simulink model "uwb_hw_cosim_kintex"  (Simulink 8.0)
settings: Solver=ode45  StartTime=0.0  StopTime=33  RelTol=1e-3
InitFcn:
  | clear
  | %set_channel;
  | load channel;
  | Int_Data_input;
StopFcn:
  | bit_to_dec_excel;
  | abc=1;
values from neighbouring files (symbols this model uses):
  bit_rate = 9.7656e5    (= 976560)    [Int_Data_input.m]
undefined symbols (not defined in the file or in its folder): rsgenpoly
libraries: commutil2 x88, simulink x53, dspmtrx3 x32, dspindex x16, commcnvcod2 x8, commblkcod2 x8, dspsigops x3, commsink2 x2, xbsIndex_r4 x1, commchan3 x1, JTAGRuntimeCosim_r4 x1
(part 1 of 5)
settings Model: Creator=minhtu  LastModifiedBy=Administrator
settings DataIOCC: SignalLoggingSaveFormat=ModelDataLogs
settings DebuggingCC: FcnCallInpInsideContextMsg=UseLocalSettings
settings CodeAppCC: CustomSymbolStrType=$N$R$M_T  InternalIdentifier=Shortened
settings GRTTargetCC: CombineOutputUpdateFcns=off  GRTInterface=on

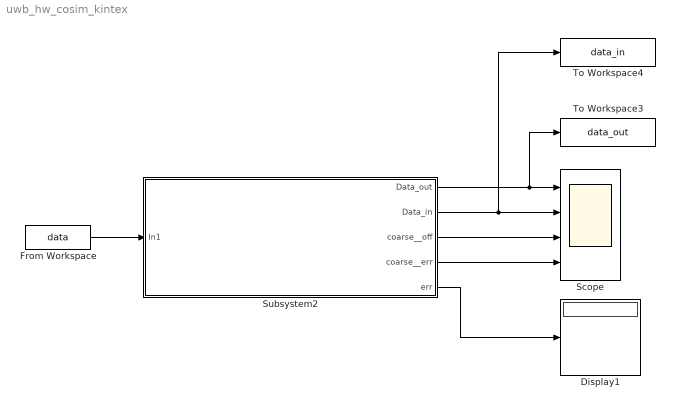
== system uwb_hw_cosim_kintex ==
  Display1 : Display
  From Workspace : FromWorkspace  VariableName=data  SampleTime=1/100
  Scope : Scope  NumInputPorts=4
      settings: YMin=0~0~1~-5  YMax=1~1~1~5  MaxDataPoints=50000000
  Subsystem2 : Subsystem
      mask Display:
      | disp('UWB_SYSTEM')
      | port_label('input',1,'data_in');
      | port_label('output',1,'data_out');
      | port_label('output',2,'data_in_delay');
      | port_label('output',3,'coarse_off');
      | port_label('output',4,'coarse_err');
      | port_label('output',5,'err');
  To Workspace3 : ToWorkspace  VariableName=data_out  SampleTime=1/100  SaveFormat=Structure
  To Workspace4 : ToWorkspace  VariableName=data_in  SampleTime=1/100  SaveFormat=Structure
  wires:
  From Workspace/1 -> Subsystem2/1(In1)
  Subsystem2/1(Data_out) -> To Workspace3/1, Scope/1
  Subsystem2/2(Data_in) -> To Workspace4/1, Scope/2
  Subsystem2/5(err) -> Display1/1
  Subsystem2/3(coarse__off) -> Scope/3
  Subsystem2/4(coarse__err) -> Scope/4

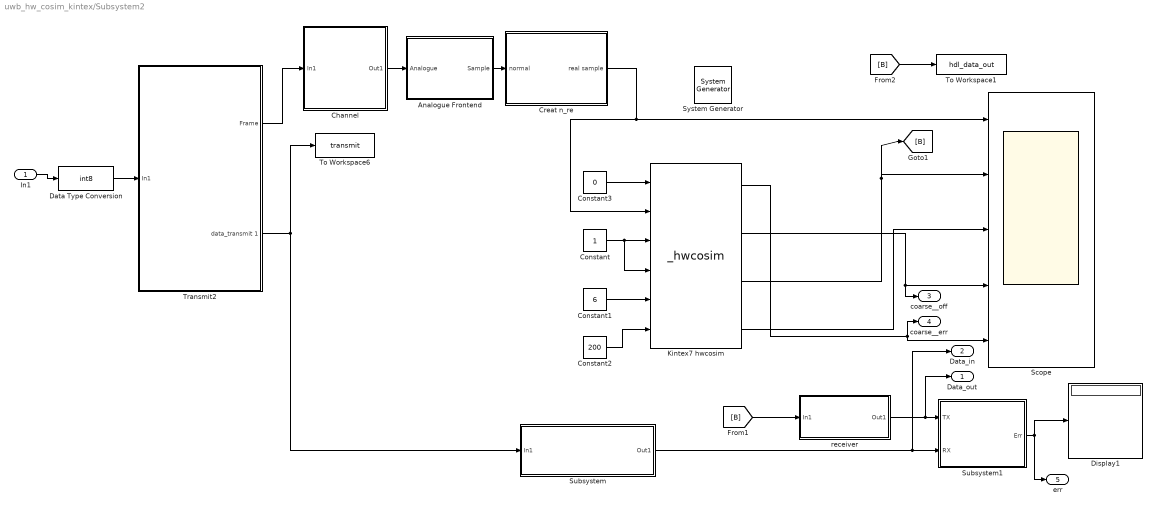
== system uwb_hw_cosim_kintex/Subsystem2 ==
  In1 : Inport
  " System Generator" : xbsIndex_r4/ System Generator  Tag=genX  xilinxfamily=kintex7  part=xc7k325t  speed=-2  package=ffg900  synthesis_tool=XST  clock_wrapper=Clock Enables  directory=./netlist  proj_type=Project Navigator  Synth_file=XST Defaults  Impl_file=ISE Defaults  testbench=off  simulink_period=3.3/31488  sysclk_period=20  dcm_input_clock_period=10  incr_netlist=off  trim_vbits=Everywhere in SubSystem  dbl_ovrd=According to Block Masks  core_generation=According to Block Masks  run_coregen=off  deprecated_control=off  eval_field=0  block_type=sysgen
  Analogue Frontend : Subsystem
  Channel : Subsystem
      mask Display: disp('CHANNEL')
  Constant : Constant
  Constant1 : Constant  Value=6
  Constant2 : Constant  Value=200
  Constant3 : Constant  Value=0
  Creat n_re : Subsystem
  Data Type Conversion : DataTypeConversion  OutDataTypeStr=int8  SampleTime=1/100
  Display1 : Display
  Kintex7 hwcosim : JTAGRuntimeCosim_r4/_hwcosim  clkSrc=Single Stepped  hasCombinationalPath=on  bitfileName=D:/z_WORKSPACE/UWB/uwb_implementation_final_kintex_final/netlist/subsystem2_cw.bit  skipConfig=off  cable=Xilinx Platform USB  speed=12 MHz  cablePort=USB21  cableParameters=xilinx_platformusb port=USB21 frequency=12000000  cableLocation=Local  shareCable=off  enable_codebug=on  savedCableParameters=xilinx_platformusb port=USB21 frequency=12000000  design_xtable=|  engineDll=JTAGCosimEngine.dll  cableWaitTime=10  bscanPos=-1  IRLengths=[]  useWaitBox=1  hasBufgmux=on  Scheme=Cosim  useCmdProc=1  hasProc=0  useImpact=0  printLogFile=0  block_type=jtagcosim
      | {
      |   'clkWrapper' => 'subsystem2_cw',
      |   'clocksGcd' => 1,
      |   'device' => 'xc7k325t-2ffg900',
      |   'ports' => {
      |     'coarse_error' => {
      |       'bd_port_index' => 0,
      |       'direction' => 'out',
      |       'icon_text' => 'coarse_error',
      |       'period' => 1,
      |       'sim_pause_trigger' => false,
      |       'type' => 'UFix_1_0',
      |       'width' => 1,
      |     },
      |     'coarse_off' => {
      |       'bd_port_index' => 1,
      |       'direction' => 'out',
      |       'icon_text' => 'coarse_off',
      |       'period' => 1,
      |       'sim_pause_trigger' => false,
      |       'type' => 'UFix_1_0',
      |       'width' => 1,
      |     },
      |     'data_out' => {
      |       'bd_port_index' => 2,
      |       'direction' => 'out',
      |       'icon_text' => 'data_out',
      |       'period' => 1,
      |       'sim_pause_trigger' => false,
      |       'type' => 'UFix_1_0',
      |       'width' => 1,
      |     },
      |     'ddph_i' => {
      |       'bd_port_index' => 0,
      |       'direction' => 'in',
      |       'icon_text' => 'ddph_i',
      |       'period' => 1,
      |       'sim_pause_trigger' => false,
      |       'type' => 'UFix_3_0',
      |       'width' => 3,
      |     },
      |     'in_data' => {
      |       'bd_port_index' => 1,
      |       'direction' => 'in',
      |       'icon_text' => 'in_data',
      |       'period' => 1,
      |       'sim_pause_trigger' => false,
      |       'type' => 'UFix_8_0',
      |       'width' => 8,
      |     },
      |     'in_rst' => {
      |       'bd_port_index' => 2,
      |       'direction' => 'in',
      |       'icon_text' => 'in_rst',
      |       'period' => 1,
      |       'sim_pause_trigger' => false,
      |       'type' => 'UFix_1_0',
      |       'width' => 1,
      |     },
      |     'in_start' => {
      |       'bd_port_index' => 3,
      |       'direction' => 'in',
      |       'icon_text' => 'in_start',
      |       'period' => 1,
      |       'sim_pause_trigger' => false,
      |       'type' => 'UFix_1_0',
      |       'width' => 1,
      |     },
      |     'psdu_en' => {
      |       'bd_port_index' => 3,
      |       'direction' => 'out',
      |       'icon_text' => 'psdu_en',
      |       'period' => 1,
      |       'sim_pause_trigger' => false,
      |       'type' => 'UFix_1_0',
      |       'width' => 1,
      |     },
      |     'sfd_threshold' => {
      |       'bd_port_index' => 4,
      |       'direction' => 'in',
      |       'icon_text' => 'sfd_threshold',
      |       'period' => 1,
      |       'sim_pause_trigger' => false,
      |       'type' => 'UFix_32_0',
      |       'width' => 32,
      |     },
      |     'sm_threshold' => {
      |       'bd_port_index' => 5,
      |       'direction' => 'in',
      |       'icon_text' => 'sm_threshold',
      |       'period' => 1,
      |       'sim_pause_trigger' => false,
      |       'type' => 'UFix_16_0',
      |       'width' => 16,
      |     },
      |   },
      |   'shared_memories' => {},
      | }
  Scope : Scope  NumInputPorts=5
      settings: TimeRange=33  YMin=0~0~0~0~0  YMax=300~1~1~1~1  MaxDataPoints=2000000
  Subsystem : Subsystem
      mask Display: disp('Delay_Data');
  Subsystem1 : Subsystem
      mask Display:
      | disp('Error Rate\n \n')
      | disp('Caculation')
      | port_label('input',1,'Rx');
      | port_label('input',2,'Tx');
      | port_label('output',1,'Err');
  To Workspace1 : ToWorkspace  VariableName=hdl_data_out  SampleTime=3.3/492  SaveFormat=Structure
  To Workspace6 : ToWorkspace  VariableName=transmit  SampleTime=3.3  SaveFormat=Structure
  Transmit2 : Subsystem
  receiver : Subsystem
      mask Display: disp('Rec_bit')
  Data_out : Outport
  Data_in : Outport  Port=2
  coarse__off : Outport  Port=3
  coarse__err : Outport  Port=4
  err : Outport  Port=5
  wires:
  Subsystem1/1(Err) -> err/1, Display1/1
  [B] -> receiver/1(In1)
  Transmit2/1(Frame) -> Channel/1(In1)
  Channel/1(Out1) -> Analogue Frontend/1(Analogue)
  Analogue Frontend/1(Sample) -> Creat n_re/1(normal)
  Kintex7 hwcosim/3 -> [B], Scope/2
  Kintex7 hwcosim/4 -> Scope/3
  Kintex7 hwcosim/2 -> coarse__off/1, Scope/4
  Kintex7 hwcosim/1 -> coarse__err/1, Scope/5
  [B] -> To Workspace1/1
  Creat n_re/1(real sample) -> Kintex7 hwcosim/2, Scope/1
  Constant3/1 -> Kintex7 hwcosim/1
  Transmit2/2(data_transmit 1) -> To Workspace6/1, Subsystem/1(In1)
  Subsystem/1(Out1) -> Data_in/1, Subsystem1/2(RX)
  Data Type Conversion/1 -> Transmit2/1(In1)
  receiver/1(Out1) -> Data_out/1, Subsystem1/1(TX)
  In1/1 -> Data Type Conversion/1
  Constant/1 -> Kintex7 hwcosim/4, Kintex7 hwcosim/3
  Constant1/1 -> Kintex7 hwcosim/5
  Constant2/1 -> Kintex7 hwcosim/6

== system uwb_hw_cosim_kintex/Subsystem2/Analogue Frontend ==
  note: Sample : 16 ns
  Analogue : Inport
  16 ns : Sum  Inputs=+  OutDataTypeStr=double
  Buffer : Buffer  N=32  TreatMby1Signals=One channel
  Product : Product  RndMeth=Zero
  Sample : Outport
  wires:
  Product/1 -> Buffer/1
  Buffer/1 -> 16 ns/1
  Analogue/1 -> Product/1, Product/2
  16 ns/1 -> Sample/1

== system uwb_hw_cosim_kintex/Subsystem2/Channel ==
  note: Channel CM1
  In1 : Inport
  AWGN Channel2 : commchan3/AWGN Channel  InputProcessing=Inherited (this choice will be removed - see release notes)  seed=0  noiseMode="Signal to noise ratio  (SNR)"  EbNodB=10  EsNodB=10  SNRdB=10  bitsPerSym=1  Ps=1  Tsym=1  variance=1
  Constant : Constant  Value=0  SampleTime=-1
  Counter Limited : simulink/Sources/Counter Limited  uplimit=10000000000000000  tsamp=3.3/1007616
  Data Type Conversion1 : DataTypeConversion  OutDataTypeStr=double
  Discrete FIR Filter : DiscreteFir  CoefSource=Input port  ProductDataTypeStr=int32  AccumDataTypeStr=int32  OutDataTypeStr=int32
  From Workspace3 : FromWorkspace  VariableName=delay  SampleTime=3.3/1007616  Interpolate=off  OutputAfterFinalValue=Cyclic repetition
  From File : FromFile  FileName=kenh.mat
  Gain1 : Gain  Gain=2^-3
  Relational Operator : RelationalOperator  Operator=<=  OutDataTypeStr=boolean
  delay_line : Subsystem
  Out1 : Outport
  wires:
  From File/1 -> Discrete FIR Filter/2
  Discrete FIR Filter/1 -> delay_line/1(data)
  Counter Limited/1 -> Relational Operator/1
  From Workspace3/1 -> Relational Operator/2
  Relational Operator/1 -> delay_line/3(sel)
  Constant/1 -> delay_line/2(loss_data)
  delay_line/1(data_out) -> AWGN Channel2/1
  In1/1 -> Gain1/1
  Data Type Conversion1/1 -> Discrete FIR Filter/1
  Gain1/1 -> Data Type Conversion1/1
  AWGN Channel2/1 -> Out1/1

== system uwb_hw_cosim_kintex/Subsystem2/Creat n_re ==
  normal : Inport
  Counter Limited2 : simulink/Sources/Counter Limited  uplimit=1000000000000  tsamp=3.3/31488
  Data Type Conversion : DataTypeConversion  OutDataTypeStr=uint8
  Delay : Constant  Value=84  OutDataTypeStr=double  SampleTime=3.3
  L_tpr4 : Constant  Value=0  VectorParams1D=off  OutDataTypeStr=double  SampleTime=-1
  Relational Operator1 : RelationalOperator  Operator=<=  OutDataTypeStr=boolean
  Remove 2 first error frames1 : Subsystem
  To Workspace : ToWorkspace  VariableName=delay  SampleTime=3.3  SaveFormat=Structure
  To Workspace3 : ToWorkspace  VariableName=Loss  SampleTime=3.3  SaveFormat=Structure
  Unbuffer : Unbuffer  SampleBasedProcessing=Same as frame based
  delay transmition : Subsystem
  n_re : Constant  Value=randi([31488,41408],1,1)  VectorParams1D=off  OutDataTypeStr=int32
  real sample : Outport
  wires:
  Relational Operator1/1 -> Remove 2 first error frames1/3(sel)
  n_re/1 -> Relational Operator1/1, To Workspace3/1
  L_tpr4/1 -> Remove 2 first error frames1/1(Zeros)
  Unbuffer/1 -> Remove 2 first error frames1/2(Sample)
  Counter Limited2/1 -> Relational Operator1/2
  Remove 2 first error frames1/1(data_out) -> delay transmition/1(data)
  normal/1 -> Unbuffer/1
  delay transmition/1(data_out) -> Data Type Conversion/1
  Delay/1 -> delay transmition/2(delay), To Workspace/1
  Data Type Conversion/1 -> real sample/1

== system uwb_hw_cosim_kintex/Subsystem2/Subsystem ==
  In1 : Inport
  Data Type Conversion2 : DataTypeConversion  OutDataTypeStr=double  SampleTime=1/100
  Delay : dspsigops/Delay  dly_unit=Samples  delay=495*2+2  ic_detail=off  dif_ic_for_ch=off  dif_ic_for_dly=off  ic=0  reset_popup=None
  Out1 : Outport
  wires:
  In1/1 -> Data Type Conversion2/1
  Data Type Conversion2/1 -> Delay/1
  Delay/1 -> Out1/1

== system uwb_hw_cosim_kintex/Subsystem2/Subsystem1 ==
  TX : Inport
  RX : Inport  Port=2
  Compare To Zero : simulink/Logic and Bit Operations/Compare To Zero  relop=>  OutDataTypeStr=uint8  ZeroCross=off
  Constant : Constant  Value=bit_rate
  Delay : dspsigops/Delay  dly_unit=Samples  delay=1  ic_detail=off  dif_ic_for_ch=off  dif_ic_for_dly=off  ic=0  reset_popup=None
  Delay1 : dspsigops/Delay  dly_unit=Samples  delay=992  ic_detail=off  dif_ic_for_ch=off  dif_ic_for_dly=off  ic=0  reset_popup=None
  Enabled Subsystem : Subsystem  TreatAsAtomicUnit=on
  Enabled Subsystem1 : Subsystem  TreatAsAtomicUnit=on
  Error Rate Calculation : commsink2/Error Rate Calculation  N=0  st_delay=992  cp_mode=Entire frame  subframe=[]  PMode=Port  WsName=ErrorVec  RsMode2=off  stop=off  numErr=100  maxBits=1e6
  Error Rate Calculation1 : commsink2/Error Rate Calculation  N=0  st_delay=992  cp_mode=Entire frame  subframe=[]  PMode=Port  WsName=ErrorVec  RsMode2=off  stop=off  numErr=100  maxBits=1e6
  Logical Operator1 : Logic  Operator=NOT  AllPortsSameDT=off  OutDataTypeStr=boolean
  Matrix Concatenate : Concatenate  Mode=Multidimensional array
  Merge : Merge
  Relational Operator : RelationalOperator  OutDataTypeStr=boolean
  Submatrix : dspmtrx3/Submatrix  RowSpan=One row  RowStartMode=Index  RowStartIndex=2  RowEndMode=Last  RowEndIndex=1  ColSpan=One column  ColStartMode=First  ColStartIndex=1  ColEndMode=Last  ColEndIndex=1
  Submatrix2 : dspmtrx3/Submatrix  RowSpan=One row  RowStartMode=Index  RowStartIndex=2  RowEndMode=Last  RowEndIndex=1  ColSpan=One column  ColStartMode=First  ColStartIndex=1  ColEndMode=Last  ColEndIndex=1
  Err : Outport
  wires:
  Error Rate Calculation/1 -> Enabled Subsystem1/1(In1), Submatrix/1
  Delay/1 -> Error Rate Calculation1/2
  Relational Operator/1 -> Compare To Zero/1
  Compare To Zero/1 -> Logical Operator1/1, Enabled Subsystem/Enable
  Enabled Subsystem1/1(Out1) -> Merge/1
  Submatrix/1 -> Relational Operator/1
  Merge/1 -> Matrix Concatenate/1
  Submatrix2/1 -> Relational Operator/2
  Enabled Subsystem/1(Out1) -> Merge/2
  TX/1 -> Error Rate Calculation1/1, Error Rate Calculation/1
  RX/1 -> Delay/1, Error Rate Calculation/2
  Logical Operator1/1 -> Enabled Subsystem1/Enable
  Error Rate Calculation1/1 -> Enabled Subsystem/1(In1), Submatrix2/1
  Constant/1 -> Delay1/1
  Delay1/1 -> Matrix Concatenate/2
  Matrix Concatenate/1 -> Err/1

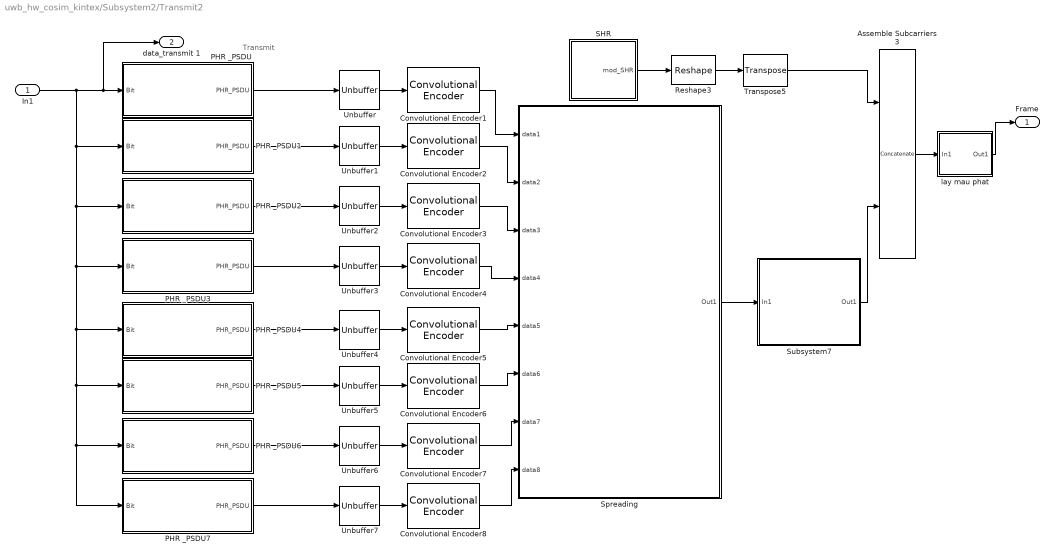
== system uwb_hw_cosim_kintex/Subsystem2/Transmit2 ==
  note: Transmit
  In1 : Inport
  Assemble Subcarriers3 : Concatenate  Mode=Multidimensional array
  Convolutional Encoder{1..8} (8 alike) : commcnvcod2/Convolutional Encoder  trellis=poly2trellis(3,[2 5])  opMode=Truncated (reset every frame)  DelayedResetAction=off  hasIniStPort=off  hasFinStPort=off  usePuncVector=off  punctureVector=[1; 1; 0; 1; 0; 1]  reset=Unused parameter value
  PHR _PSDU : Subsystem
  PHR _PSDU1 : Subsystem
  PHR _PSDU2 : Subsystem
  PHR _PSDU3 : Subsystem
  PHR _PSDU4 : Subsystem
  PHR _PSDU5 : Subsystem
  PHR _PSDU6 : Subsystem
  PHR _PSDU7 : Subsystem
  Reshape3 : Reshape  OutputDimensionality=Customize  OutputDimensions=[5,5952*32]
  SHR : Subsystem
  Spreading : Subsystem
  Subsystem7 : Subsystem
      mask Display: disp('data trc SHR');
  Transpose5 : dspmtrx3/Transpose  Hermitian=off  overflowFlag=off
  Unbuffer{,1..7} (8 alike) : Unbuffer
  lay mau phat : Subsystem
      mask Display: disp('sample')
  Frame : Outport
  data_transmit 1 : Outport  Port=2
  wires:
  Spreading/1(Out1) -> Subsystem7/1(In1)
  Convolutional Encoder4/1 -> Spreading/4(data4)
  Convolutional Encoder3/1 -> Spreading/3(data3)
  Convolutional Encoder2/1 -> Spreading/2(data2)
  Convolutional Encoder1/1 -> Spreading/1(data1)
  Unbuffer3/1 -> Convolutional Encoder4/1
  PHR _PSDU3/1(PHR_PSDU) -> Unbuffer3/1
  Unbuffer2/1 -> Convolutional Encoder3/1
  PHR _PSDU2/1(PHR_PSDU) -> Unbuffer2/1
  Unbuffer1/1 -> Convolutional Encoder2/1
  PHR _PSDU1/1(PHR_PSDU) -> Unbuffer1/1
  lay mau phat/1(Out1) -> Frame/1
  Transpose5/1 -> Assemble Subcarriers3/1
  SHR/1(mod_SHR) -> Reshape3/1
  Reshape3/1 -> Transpose5/1
  Assemble Subcarriers3/1 -> lay mau phat/1(In1)
  Subsystem7/1(Out1) -> Assemble Subcarriers3/2
  Unbuffer/1 -> Convolutional Encoder1/1
  PHR _PSDU/1(PHR_PSDU) -> Unbuffer/1
  Unbuffer7/1 -> Convolutional Encoder8/1
  PHR _PSDU7/1(PHR_PSDU) -> Unbuffer7/1
  In1/1 -> PHR _PSDU6/1(Bit), PHR _PSDU7/1(Bit), PHR _PSDU5/1(Bit), PHR _PSDU4/1(Bit), PHR _PSDU3/1(Bit), PHR _PSDU2/1(Bit), PHR _PSDU1/1(Bit), data_transmit 1/1, PHR _PSDU/1(Bit)
  Unbuffer6/1 -> Convolutional Encoder7/1
  PHR _PSDU6/1(PHR_PSDU) -> Unbuffer6/1
  Unbuffer5/1 -> Convolutional Encoder6/1
  PHR _PSDU5/1(PHR_PSDU) -> Unbuffer5/1
  Unbuffer4/1 -> Convolutional Encoder5/1
  PHR _PSDU4/1(PHR_PSDU) -> Unbuffer4/1
  Convolutional Encoder5/1 -> Spreading/5(data5)
  Convolutional Encoder6/1 -> Spreading/6(data6)
  Convolutional Encoder7/1 -> Spreading/7(data7)
  Convolutional Encoder8/1 -> Spreading/8(data8)

== system uwb_hw_cosim_kintex/Subsystem2/receiver ==
  In1 : Inport
  Buffer : Buffer  N=492  TreatMby1Signals=One channel
  Data Type Conversion2 : DataTypeConversion  OutDataTypeStr=double  SampleTime=3.3/492
  Submatrix : dspmtrx3/Submatrix  RowSpan=Range of rows  RowStartMode=Index  RowStartIndex=113  RowEndMode=Index  RowEndIndex=442  ColSpan=One column  ColStartMode=First  ColStartIndex=1  ColEndMode=Last  ColEndIndex=1
  Unbuffer : Unbuffer  SampleBasedProcessing=Same as frame based
  Out1 : Outport
  wires:
  In1/1 -> Data Type Conversion2/1
  Unbuffer/1 -> Out1/1
  Submatrix/1 -> Unbuffer/1
  Buffer/1 -> Submatrix/1
  Data Type Conversion2/1 -> Buffer/1

== system uwb_hw_cosim_kintex/Subsystem2/Channel/delay_line ==
  data : Inport
  loss_data : Inport  Port=2
  sel : Inport  Port=3
  Compare To Zero : simulink/Logic and Bit Operations/Compare To Zero  relop===  OutDataTypeStr=uint8  ZeroCross=off
  Enabled Subsystem : Subsystem  TreatAsAtomicUnit=on
  Enabled Subsystem1 : Subsystem  TreatAsAtomicUnit=on
  Logical Operator : Logic  Operator=NOT  AllPortsSameDT=off  OutDataTypeStr=boolean
  Merge : Merge
  data_out : Outport
  wires:
  loss_data/1 -> Enabled Subsystem/1(In1)
  Merge/1 -> data_out/1
  sel/1 -> Compare To Zero/1
  data/1 -> Enabled Subsystem1/1(In1)
  Compare To Zero/1 -> Logical Operator/1, Enabled Subsystem1/Enable
  Enabled Subsystem1/1(Out1) -> Merge/1
  Enabled Subsystem/1(Out1) -> Merge/2
  Logical Operator/1 -> Enabled Subsystem/Enable

== system uwb_hw_cosim_kintex/Subsystem2/Creat n_re/Remove 2 first error frames1 ==
  Zeros : Inport
  Sample : Inport  Port=2
  sel : Inport  Port=3
  Compare To Zero : simulink/Logic and Bit Operations/Compare To Zero  relop===  OutDataTypeStr=uint8  ZeroCross=off
  Enabled Subsystem : Subsystem  TreatAsAtomicUnit=on
  Enabled Subsystem1 : Subsystem  TreatAsAtomicUnit=on
  Logical Operator : Logic  Operator=NOT  AllPortsSameDT=off  OutDataTypeStr=boolean
  Merge : Merge
  data_out : Outport
  wires:
  Sample/1 -> Enabled Subsystem/1(In1)
  Merge/1 -> data_out/1
  sel/1 -> Compare To Zero/1
  Zeros/1 -> Enabled Subsystem1/1(In1)
  Compare To Zero/1 -> Logical Operator/1, Enabled Subsystem1/Enable
  Enabled Subsystem1/1(Out1) -> Merge/1
  Enabled Subsystem/1(Out1) -> Merge/2
  Logical Operator/1 -> Enabled Subsystem/Enable

== system uwb_hw_cosim_kintex/Subsystem2/Creat n_re/delay transmition ==
  note: tre hang nghin k dung den
  data : Inport
  delay : Inport  Port=2
  Display{,1..5} (6 alike) : Display
  Truyen Tre : Subsystem
  Truyen Tre chuc : Subsystem
  Truyen Tre don vi : Subsystem
  Truyen Tre tram : Subsystem
  hang chuc : Subsystem
  hang don vi : Subsystem
  hang nghin : Subsystem
  hang tram : Subsystem
  tach delay : Subsystem
  data_out : Outport
  wires:
  hang nghin/1(Out1) -> Truyen Tre/2(In1)
  hang nghin/2(Out2) -> Truyen Tre/3(In2)
  data/1 -> hang nghin/1(In1)
  Truyen Tre/1(data) -> hang tram/1(In1)
  Truyen Tre don vi/1(data) -> data_out/1
  delay/1 -> tach delay/1(delay), Display1/1
  Truyen Tre tram/1(data) -> hang chuc/1(In1)
  Truyen Tre chuc/1(data) -> hang don vi/1(In1)
  tach delay/2(chuc) -> Truyen Tre chuc/1(case), Display3/1
  tach delay/4(Nghin) -> Truyen Tre/1(case), Display5/1
  tach delay/3(Tram) -> Truyen Tre tram/1(case), Display2/1
  tach delay/1(donvi) -> Truyen Tre don vi/1(case), Display4/1
  tach delay/5(tre kenh) -> Display/1
  hang tram/2(Out2) -> Truyen Tre tram/2(In2)
  hang tram/3(Out3) -> Truyen Tre tram/3(In3)
  hang tram/4(Out4) -> Truyen Tre tram/4(In4)
  hang tram/5(Out5) -> Truyen Tre tram/5(In5)
  hang tram/6(Out6) -> Truyen Tre tram/6(In6)
  hang tram/7(Out7) -> Truyen Tre tram/7(In7)
  hang tram/8(Out8) -> Truyen Tre tram/8(In8)
  hang tram/9(Out9) -> Truyen Tre tram/9(In9)
  hang tram/10(Out10) -> Truyen Tre tram/10(In10)
  hang tram/1(Out1) -> Truyen Tre tram/11(In11)
  hang chuc/2(Out2) -> Truyen Tre chuc/2(In2)
  hang chuc/3(Out3) -> Truyen Tre chuc/3(In3)
  hang chuc/4(Out4) -> Truyen Tre chuc/4(In4)
  hang chuc/5(Out5) -> Truyen Tre chuc/5(In5)
  hang chuc/6(Out6) -> Truyen Tre chuc/6(In6)
  hang chuc/7(Out7) -> Truyen Tre chuc/7(In7)
  hang chuc/8(Out8) -> Truyen Tre chuc/8(In8)
  hang chuc/9(Out9) -> Truyen Tre chuc/9(In9)
  hang chuc/10(Out10) -> Truyen Tre chuc/10(In10)
  hang chuc/1(Out1) -> Truyen Tre chuc/11(In11)
  hang don vi/2(Out2) -> Truyen Tre don vi/2(In2)
  hang don vi/3(Out3) -> Truyen Tre don vi/3(In3)
  hang don vi/4(Out4) -> Truyen Tre don vi/4(In4)
  hang don vi/5(Out5) -> Truyen Tre don vi/5(In5)
  hang don vi/6(Out6) -> Truyen Tre don vi/6(In6)
  hang don vi/7(Out7) -> Truyen Tre don vi/7(In7)
  hang don vi/8(Out8) -> Truyen Tre don vi/8(In8)
  hang don vi/9(Out9) -> Truyen Tre don vi/9(In9)
  hang don vi/10(Out10) -> Truyen Tre don vi/10(In10)
  hang don vi/1(Out1) -> Truyen Tre don vi/11(In11)

== system uwb_hw_cosim_kintex/Subsystem2/Subsystem1/Enabled Subsystem ==
  In1 : Inport
  Enable : EnablePort  PropagateVarSize=During execution
  Out1 : Outport
  wires:
  In1/1 -> Out1/1

== system uwb_hw_cosim_kintex/Subsystem2/Subsystem1/Enabled Subsystem1 ==
  In1 : Inport
  Enable : EnablePort  PropagateVarSize=During execution
  Out1 : Outport
  wires:
  In1/1 -> Out1/1

== system uwb_hw_cosim_kintex/Subsystem2/Transmit2/PHR _PSDU ==
  Bit : Inport
  Assemble Subcarriers : Concatenate  Mode=Multidimensional array
  Assemble Subcarriers1 : Concatenate  NumInputs=3  Mode=Multidimensional array
  Buffer 330bit : Buffer  N=330
  CONST : Constant  Value=[0 0]  VectorParams1D=off  OutDataTypeStr=int8  SampleTime=1  FramePeriod=3.3
      settings: SamplingMode=Frame based
  General PHR1 : Subsystem
  Reshape : Reshape  OutputDimensionality=Column vector (2-D)  OutputDimensions=[10,1]
  Reshape1 : Reshape  OutputDimensionality=Column vector (2-D)  OutputDimensions=[10,1]
  Subsystem6 : Subsystem
      mask Display:
      | disp('Reed Solomon.E');
      | port_label('input',1,'bit_in');
      | port_label('output',1,'bit_out');
  PHR_PSDU : Outport
  wires:
  Assemble Subcarriers1/1 -> PHR_PSDU/1
  Bit/1 -> Subsystem6/1(In1), Buffer 330bit/1
  Buffer 330bit/1 -> Assemble Subcarriers/1
  Assemble Subcarriers/1 -> Assemble Subcarriers1/2
  General PHR1/1(PHR) -> Reshape/1
  Reshape/1 -> Assemble Subcarriers1/1
  CONST/1 -> Reshape1/1
  Reshape1/1 -> Assemble Subcarriers1/3
  Subsystem6/1(Out1) -> Assemble Subcarriers/2

== system uwb_hw_cosim_kintex/Subsystem2/Transmit2/PHR _PSDU1 ==
  Bit : Inport
  Assemble Subcarriers : Concatenate  Mode=Multidimensional array
  Assemble Subcarriers1 : Concatenate  NumInputs=3  Mode=Multidimensional array
  Buffer 330bit : Buffer  N=330
  CONST : Constant  Value=[0 0]  VectorParams1D=off  OutDataTypeStr=int8  SampleTime=1  FramePeriod=3.3
      settings: SamplingMode=Frame based
  General PHR1 : Subsystem
  Reshape : Reshape  OutputDimensionality=Column vector (2-D)  OutputDimensions=[10,1]
  Reshape1 : Reshape  OutputDimensionality=Column vector (2-D)  OutputDimensions=[10,1]
  Subsystem6 : Subsystem
      mask Display:
      | disp('Reed Solomon.E');
      | port_label('input',1,'bit_in');
      | port_label('output',1,'bit_out');
  PHR_PSDU : Outport
  wires:
  Subsystem6/1(Out1) -> Assemble Subcarriers/2
  Reshape1/1 -> Assemble Subcarriers1/3
  CONST/1 -> Reshape1/1
  Reshape/1 -> Assemble Subcarriers1/1
  General PHR1/1(PHR) -> Reshape/1
  Assemble Subcarriers/1 -> Assemble Subcarriers1/2
  Buffer 330bit/1 -> Assemble Subcarriers/1
  Bit/1 -> Buffer 330bit/1, Subsystem6/1(In1)
  Assemble Subcarriers1/1 -> PHR_PSDU/1

== system uwb_hw_cosim_kintex/Subsystem2/Transmit2/PHR _PSDU2 ==
  Bit : Inport
  Assemble Subcarriers : Concatenate  Mode=Multidimensional array
  Assemble Subcarriers1 : Concatenate  NumInputs=3  Mode=Multidimensional array
  Buffer 330bit : Buffer  N=330
  CONST : Constant  Value=[0 0]  VectorParams1D=off  OutDataTypeStr=int8  SampleTime=1  FramePeriod=3.3
      settings: SamplingMode=Frame based
  General PHR1 : Subsystem
  Reshape : Reshape  OutputDimensionality=Column vector (2-D)  OutputDimensions=[10,1]
  Reshape1 : Reshape  OutputDimensionality=Column vector (2-D)  OutputDimensions=[10,1]
  Subsystem6 : Subsystem
      mask Display:
      | disp('Reed Solomon.E');
      | port_label('input',1,'bit_in');
      | port_label('output',1,'bit_out');
  PHR_PSDU : Outport
  wires:
  Assemble Subcarriers1/1 -> PHR_PSDU/1
  Bit/1 -> Subsystem6/1(In1), Buffer 330bit/1
  Buffer 330bit/1 -> Assemble Subcarriers/1
  Assemble Subcarriers/1 -> Assemble Subcarriers1/2
  General PHR1/1(PHR) -> Reshape/1
  Reshape/1 -> Assemble Subcarriers1/1
  CONST/1 -> Reshape1/1
  Reshape1/1 -> Assemble Subcarriers1/3
  Subsystem6/1(Out1) -> Assemble Subcarriers/2

== system uwb_hw_cosim_kintex/Subsystem2/Transmit2/PHR _PSDU3 ==
  Bit : Inport
  Assemble Subcarriers : Concatenate  Mode=Multidimensional array
  Assemble Subcarriers1 : Concatenate  NumInputs=3  Mode=Multidimensional array
  Buffer 330bit : Buffer  N=330
  CONST : Constant  Value=[0 0]  VectorParams1D=off  OutDataTypeStr=int8  SampleTime=1  FramePeriod=3.3
      settings: SamplingMode=Frame based
  General PHR1 : Subsystem
  Reshape : Reshape  OutputDimensionality=Column vector (2-D)  OutputDimensions=[10,1]
  Reshape1 : Reshape  OutputDimensionality=Column vector (2-D)  OutputDimensions=[10,1]
  Subsystem6 : Subsystem
      mask Display:
      | disp('Reed Solomon.E');
      | port_label('input',1,'bit_in');
      | port_label('output',1,'bit_out');
  PHR_PSDU : Outport
  wires:
  Subsystem6/1(Out1) -> Assemble Subcarriers/2
  Reshape1/1 -> Assemble Subcarriers1/3
  CONST/1 -> Reshape1/1
  Reshape/1 -> Assemble Subcarriers1/1
  General PHR1/1(PHR) -> Reshape/1
  Assemble Subcarriers/1 -> Assemble Subcarriers1/2
  Buffer 330bit/1 -> Assemble Subcarriers/1
  Bit/1 -> Buffer 330bit/1, Subsystem6/1(In1)
  Assemble Subcarriers1/1 -> PHR_PSDU/1

== system uwb_hw_cosim_kintex/Subsystem2/Transmit2/PHR _PSDU4 ==
  Bit : Inport
  Assemble Subcarriers : Concatenate  Mode=Multidimensional array
  Assemble Subcarriers1 : Concatenate  NumInputs=3  Mode=Multidimensional array
  Buffer 330bit : Buffer  N=330
  CONST : Constant  Value=[0 0]  VectorParams1D=off  OutDataTypeStr=int8  SampleTime=1  FramePeriod=3.3
      settings: SamplingMode=Frame based
  General PHR1 : Subsystem
  Reshape : Reshape  OutputDimensionality=Column vector (2-D)  OutputDimensions=[10,1]
  Reshape1 : Reshape  OutputDimensionality=Column vector (2-D)  OutputDimensions=[10,1]
  Subsystem6 : Subsystem
      mask Display:
      | disp('Reed Solomon.E');
      | port_label('input',1,'bit_in');
      | port_label('output',1,'bit_out');
  PHR_PSDU : Outport
  wires:
  Subsystem6/1(Out1) -> Assemble Subcarriers/2
  Reshape1/1 -> Assemble Subcarriers1/3
  CONST/1 -> Reshape1/1
  Reshape/1 -> Assemble Subcarriers1/1
  General PHR1/1(PHR) -> Reshape/1
  Assemble Subcarriers/1 -> Assemble Subcarriers1/2
  Buffer 330bit/1 -> Assemble Subcarriers/1
  Bit/1 -> Buffer 330bit/1, Subsystem6/1(In1)
  Assemble Subcarriers1/1 -> PHR_PSDU/1

== system uwb_hw_cosim_kintex/Subsystem2/Transmit2/PHR _PSDU5 ==
  Bit : Inport
  Assemble Subcarriers : Concatenate  Mode=Multidimensional array
  Assemble Subcarriers1 : Concatenate  NumInputs=3  Mode=Multidimensional array
  Buffer 330bit : Buffer  N=330
  CONST : Constant  Value=[0 0]  VectorParams1D=off  OutDataTypeStr=int8  SampleTime=1  FramePeriod=3.3
      settings: SamplingMode=Frame based
  General PHR1 : Subsystem
  Reshape : Reshape  OutputDimensionality=Column vector (2-D)  OutputDimensions=[10,1]
  Reshape1 : Reshape  OutputDimensionality=Column vector (2-D)  OutputDimensions=[10,1]
  Subsystem6 : Subsystem
      mask Display:
      | disp('Reed Solomon.E');
      | port_label('input',1,'bit_in');
      | port_label('output',1,'bit_out');
  PHR_PSDU : Outport
  wires:
  Assemble Subcarriers1/1 -> PHR_PSDU/1
  Bit/1 -> Subsystem6/1(In1), Buffer 330bit/1
  Buffer 330bit/1 -> Assemble Subcarriers/1
  Assemble Subcarriers/1 -> Assemble Subcarriers1/2
  General PHR1/1(PHR) -> Reshape/1
  Reshape/1 -> Assemble Subcarriers1/1
  CONST/1 -> Reshape1/1
  Reshape1/1 -> Assemble Subcarriers1/3
  Subsystem6/1(Out1) -> Assemble Subcarriers/2

== system uwb_hw_cosim_kintex/Subsystem2/Transmit2/PHR _PSDU6 ==
  Bit : Inport
  Assemble Subcarriers : Concatenate  Mode=Multidimensional array
  Assemble Subcarriers1 : Concatenate  NumInputs=3  Mode=Multidimensional array
  Buffer 330bit : Buffer  N=330
  CONST : Constant  Value=[0 0]  VectorParams1D=off  OutDataTypeStr=int8  SampleTime=1  FramePeriod=3.3
      settings: SamplingMode=Frame based
  General PHR1 : Subsystem
  Reshape : Reshape  OutputDimensionality=Column vector (2-D)  OutputDimensions=[10,1]
  Reshape1 : Reshape  OutputDimensionality=Column vector (2-D)  OutputDimensions=[10,1]
  Subsystem6 : Subsystem
      mask Display:
      | disp('Reed Solomon.E');
      | port_label('input',1,'bit_in');
      | port_label('output',1,'bit_out');
  PHR_PSDU : Outport
  wires:
  Subsystem6/1(Out1) -> Assemble Subcarriers/2
  Reshape1/1 -> Assemble Subcarriers1/3
  CONST/1 -> Reshape1/1
  Reshape/1 -> Assemble Subcarriers1/1
  General PHR1/1(PHR) -> Reshape/1
  Assemble Subcarriers/1 -> Assemble Subcarriers1/2
  Buffer 330bit/1 -> Assemble Subcarriers/1
  Bit/1 -> Buffer 330bit/1, Subsystem6/1(In1)
  Assemble Subcarriers1/1 -> PHR_PSDU/1

== system uwb_hw_cosim_kintex/Subsystem2/Transmit2/PHR _PSDU7 ==
  Bit : Inport
  Assemble Subcarriers : Concatenate  Mode=Multidimensional array
  Assemble Subcarriers1 : Concatenate  NumInputs=3  Mode=Multidimensional array
  Buffer 330bit : Buffer  N=330
  CONST : Constant  Value=[0 0]  VectorParams1D=off  OutDataTypeStr=int8  SampleTime=1  FramePeriod=3.3
      settings: SamplingMode=Frame based
  General PHR1 : Subsystem
  Reshape : Reshape  OutputDimensionality=Column vector (2-D)  OutputDimensions=[10,1]
  Reshape1 : Reshape  OutputDimensionality=Column vector (2-D)  OutputDimensions=[10,1]
  Subsystem6 : Subsystem
      mask Display:
      | disp('Reed Solomon.E');
      | port_label('input',1,'bit_in');
      | port_label('output',1,'bit_out');
  PHR_PSDU : Outport
  wires:
  Assemble Subcarriers1/1 -> PHR_PSDU/1
  Bit/1 -> Subsystem6/1(In1), Buffer 330bit/1
  Buffer 330bit/1 -> Assemble Subcarriers/1
  Assemble Subcarriers/1 -> Assemble Subcarriers1/2
  General PHR1/1(PHR) -> Reshape/1
  Reshape/1 -> Assemble Subcarriers1/1
  CONST/1 -> Reshape1/1
  Reshape1/1 -> Assemble Subcarriers1/3
  Subsystem6/1(Out1) -> Assemble Subcarriers/2

== system uwb_hw_cosim_kintex/Subsystem2/Transmit2/SHR ==
  note: L = 64, Nsync = 16, Nsfd = 8
  Ci1 : Constant  Value=[1 1 0 0 1 0 0 -1 -1 -1 1 -1 0 1 1 -1 0 0 0 1 0 1 0 -1 1 0 1 0 0 0 0]  VectorParams1D=off  OutDataTypeStr=int8
  Kron : MATLAB Function  TreatAsAtomicUnit=on
  Kron1 : MATLAB Function  TreatAsAtomicUnit=on
  Kron2 : MATLAB Function  TreatAsAtomicUnit=on
  Kron3 : MATLAB Function  TreatAsAtomicUnit=on
  Matrix : Concatenate  Mode=Multidimensional array  ConcatenateDimension=2
  Nsfd = 8 : Constant  Value=[0 1 0 -1 1 0 0 -1]  VectorParams1D=off  OutDataTypeStr=int8
  Nsync = 16 : Constant  Value=ones(1,16)  VectorParams1D=off  OutDataTypeStr=int8
  deltaL1 : Constant  Value=[1 zeros(1,63)]  VectorParams1D=off  OutDataTypeStr=int8
  p : Constant  Value=[-0.0022 -0.0103 -0.0386 -0.1133 -0.2542 -0.4160 -0.4388 -0.1363 0.4543 0.9559 0.9559 0.4543 -0.1363 -0.4388 -0.4160 -0.2542 -0.1133 -0.0386 -0.0103 -0.0022]*2^6  VectorParams1D=off  OutDataTypeStr=int8
      mask Display: disp('xung P')
  mod_SHR : Outport
  wires:
  Kron3/1(mod_SHR) -> mod_SHR/1
  p/1 -> Kron3/2(p)
  Matrix/1 -> Kron3/1(SHR)
  Kron/1(Si) -> Kron1/2(Si), Kron2/2(Si)
  Ci1/1 -> Kron/1(Ci)
  deltaL1/1 -> Kron/2(deltaL)
  Nsync = 16/1 -> Kron1/1(Nsync)
  Nsfd = 8/1 -> Kron2/1(Nsfd)
  Kron2/1(SFD) -> Matrix/2
  Kron1/1(SYNC) -> Matrix/1

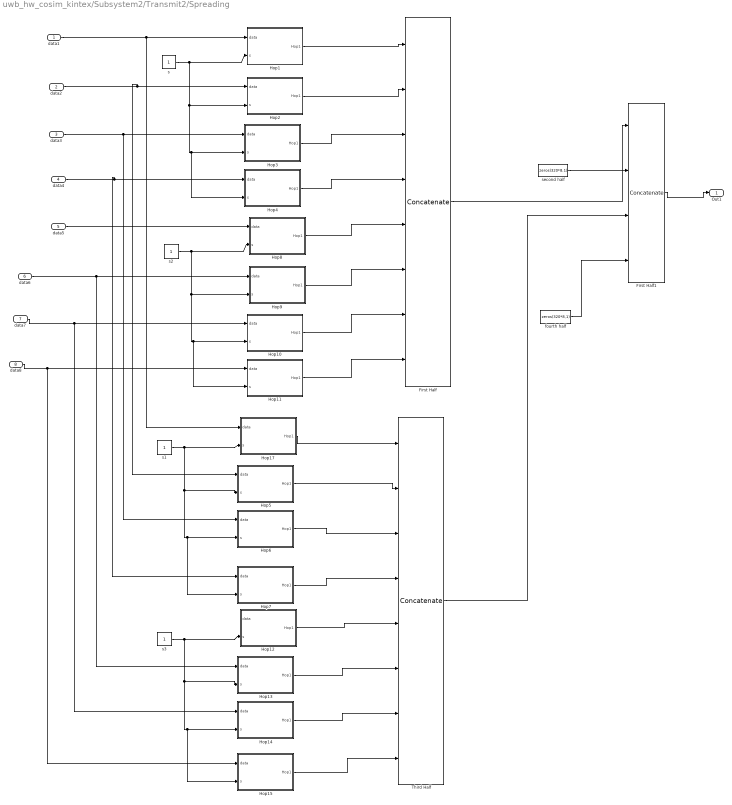
== system uwb_hw_cosim_kintex/Subsystem2/Transmit2/Spreading ==
  data1 : Inport
  data2 : Inport  Port=2
  data3 : Inport  Port=3
  data4 : Inport  Port=4
  data5 : Inport  Port=5
  data6 : Inport  Port=6
  data7 : Inport  Port=7
  data8 : Inport  Port=8
  First Half : Concatenate  NumInputs=8  Mode=Multidimensional array
  First Half1 : Concatenate  NumInputs=4  Mode=Multidimensional array
  Hop1 : Subsystem
  Hop10 : Subsystem
  Hop11 : Subsystem
  Hop12 : Subsystem
  Hop13 : Subsystem
  Hop14 : Subsystem
  Hop15 : Subsystem
  Hop17 : Subsystem
  Hop2 : Subsystem
  Hop3 : Subsystem
  Hop4 : Subsystem
  Hop5 : Subsystem
  Hop6 : Subsystem
  Hop7 : Subsystem
  Hop8 : Subsystem
  Hop9 : Subsystem
  Third Half : Concatenate  NumInputs=8  Mode=Multidimensional array
  fourth half : Constant  Value=zeros(320*8,1)  VectorParams1D=off  OutDataTypeStr=int8
      settings: SamplingMode=Frame based
  s{,1..3} (4 alike) : Constant  OutDataTypeStr=int8  SampleTime=3.3/(399*16)
  second half : Constant  Value=zeros(320*8,1)  VectorParams1D=off  OutDataTypeStr=int8
      settings: SamplingMode=Frame based
  Out1 : Outport
  wires:
  First Half1/1 -> Out1/1
  fourth half/1 -> First Half1/4
  second half/1 -> First Half1/2
  Third Half/1 -> First Half1/3
  First Half/1 -> First Half1/1
  Hop7/1(Hop1) -> Third Half/4
  Hop6/1(Hop1) -> Third Half/3
  Hop5/1(Hop1) -> Third Half/2
  s1/1 -> Hop17/2(s), Hop5/2(s), Hop7/2(s), Hop6/2(s)
  Hop17/1(Hop1) -> Third Half/1
  data4/1 -> Hop4/1(data), Hop7/1(data)
  data3/1 -> Hop3/1(data), Hop6/1(data)
  data2/1 -> Hop2/1(data), Hop5/1(data)
  Hop4/1(Hop1) -> First Half/4
  Hop3/1(Hop1) -> First Half/3
  Hop2/1(Hop1) -> First Half/2
  s/1 -> Hop2/2(s), Hop4/2(s), Hop3/2(s), Hop1/2(s)
  Hop1/1(Hop1) -> First Half/1
  data1/1 -> Hop1/1(data), Hop17/1(data)
  data8/1 -> Hop11/1(data), Hop15/1(data)
  data7/1 -> Hop10/1(data), Hop14/1(data)
  data6/1 -> Hop9/1(data), Hop13/1(data)
  s2/1 -> Hop8/2(s), Hop10/2(s), Hop11/2(s), Hop9/2(s)
  data5/1 -> Hop8/1(data)
  Hop8/1(Hop1) -> First Half/5
  Hop9/1(Hop1) -> First Half/6
  Hop10/1(Hop1) -> First Half/7
  Hop11/1(Hop1) -> First Half/8
  s3/1 -> Hop14/2(s), Hop15/2(s), Hop13/2(s), Hop12/2(s)
  Hop12/1(Hop1) -> Third Half/5
  Hop13/1(Hop1) -> Third Half/6
  Hop14/1(Hop1) -> Third Half/7
  Hop15/1(Hop1) -> Third Half/8

== system uwb_hw_cosim_kintex/Subsystem2/Transmit2/Subsystem7 ==
  In1 : Inport
  Buffer 48bit2 : Buffer  N=399
  Reshape5 : Reshape  OutputDimensionality=Customize  OutputDimensions=[5,32*25536]
  Transpose1 : dspmtrx3/Transpose  Hermitian=off  overflowFlag=off
  Transpose2 : dspmtrx3/Transpose  Hermitian=off  overflowFlag=off
  Transpose3 : dspmtrx3/Transpose  Hermitian=off  overflowFlag=off
  Out1 : Outport
  wires:
  Transpose1/1 -> Out1/1
  In1/1 -> Transpose2/1
  Reshape5/1 -> Transpose1/1
  Transpose3/1 -> Reshape5/1
  Transpose2/1 -> Buffer 48bit2/1
  Buffer 48bit2/1 -> Transpose3/1

== system uwb_hw_cosim_kintex/Subsystem2/Transmit2/lay mau phat ==
  In1 : Inport
  Buffer 48bit1 : Buffer  N=1
  Selector : Selector  InputPortWidth=5  IndexOptions=Index vector (dialog)  Indices=[1]  OutputSizes=1
  Transpose3 : dspmtrx3/Transpose  Hermitian=off  overflowFlag=off
  Out1 : Outport
  wires:
  Buffer 48bit1/1 -> Transpose3/1
  Transpose3/1 -> Selector/1
  In1/1 -> Buffer 48bit1/1
  Selector/1 -> Out1/1

== system uwb_hw_cosim_kintex/Subsystem2/Channel/delay_line/Enabled Subsystem ==
  In1 : Inport
  Enable : EnablePort  PropagateVarSize=During execution
  Out1 : Outport
  wires:
  In1/1 -> Out1/1

== system uwb_hw_cosim_kintex/Subsystem2/Channel/delay_line/Enabled Subsystem1 ==
  In1 : Inport
  Enable : EnablePort  PropagateVarSize=During execution
  Out1 : Outport
  wires:
  In1/1 -> Out1/1

== system uwb_hw_cosim_kintex/Subsystem2/Creat n_re/Remove 2 first error frames1/Enabled Subsystem ==
  In1 : Inport
  Enable : EnablePort  PropagateVarSize=During execution
  Out1 : Outport
  wires:
  In1/1 -> Out1/1

== system uwb_hw_cosim_kintex/Subsystem2/Creat n_re/Remove 2 first error frames1/Enabled Subsystem1 ==
  In1 : Inport
  Enable : EnablePort  PropagateVarSize=During execution
  Out1 : Outport
  wires:
  In1/1 -> Out1/1

== system uwb_hw_cosim_kintex/Subsystem2/Creat n_re/delay transmition/Truyen Tre ==
  case : Inport
  In1 : Inport  Port=2
  In2 : Inport  Port=3
  Merge : Merge
  Switch Case : SwitchCase
  Switch Case Action Subsystem : Subsystem  TreatAsAtomicUnit=on
      mask Display: disp('case 1')
  Switch Case Action Subsystem1 : Subsystem  TreatAsAtomicUnit=on
      mask Display: disp('case 2')
  data : Outport
  wires:
  case/1 -> Switch Case/1
  Merge/1 -> data/1
  Switch Case Action Subsystem/1(Out1) -> Merge/1
  Switch Case/1 -> Switch Case Action Subsystem/Action
  Switch Case Action Subsystem1/1(Out1) -> Merge/2
  Switch Case/2 -> Switch Case Action Subsystem1/Action
  In1/1 -> Switch Case Action Subsystem/1(In1)
  In2/1 -> Switch Case Action Subsystem1/1(In1)

== system uwb_hw_cosim_kintex/Subsystem2/Creat n_re/delay transmition/Truyen Tre chuc ==
  case : Inport
  In2 : Inport  Port=2
  In3 : Inport  Port=3
  In4 : Inport  Port=4
  In5 : Inport  Port=5
  In6 : Inport  Port=6
  In7 : Inport  Port=7
  In8 : Inport  Port=8
  In9 : Inport  Port=9
  In10 : Inport  Port=10
  In11 : Inport  Port=11
  Merge : Merge  Inputs=10
  Switch Case : SwitchCase  CaseConditions={1,2,3,4,5,6,7,8,9}
  Switch Case Action Subsystem : Subsystem  TreatAsAtomicUnit=on
      mask Display: disp('case 1')
  Switch Case Action Subsystem1 : Subsystem  TreatAsAtomicUnit=on
      mask Display: disp('case 2')
  Switch Case Action Subsystem2 : Subsystem  TreatAsAtomicUnit=on
      mask Display: disp('case 3')
  Switch Case Action Subsystem3 : Subsystem  TreatAsAtomicUnit=on
      mask Display: disp('case 4')
  Switch Case Action Subsystem4 : Subsystem  TreatAsAtomicUnit=on
      mask Display: disp('case 5')
  Switch Case Action Subsystem5 : Subsystem  TreatAsAtomicUnit=on
      mask Display: disp('case 6')
  Switch Case Action Subsystem6 : Subsystem  TreatAsAtomicUnit=on
      mask Display: disp('case 8')
  Switch Case Action Subsystem7 : Subsystem  TreatAsAtomicUnit=on
      mask Display: disp('case 7')
  Switch Case Action Subsystem8 : Subsystem  TreatAsAtomicUnit=on
      mask Display: disp('case 9')
  Switch Case Action Subsystem9 : Subsystem  TreatAsAtomicUnit=on
      mask Display: disp('case 10')
  data : Outport
  wires:
  In11/1 -> Switch Case Action Subsystem9/1(In1)
  In10/1 -> Switch Case Action Subsystem8/1(In1)
  In9/1 -> Switch Case Action Subsystem6/1(In1)
  In8/1 -> Switch Case Action Subsystem7/1(In1)
  In7/1 -> Switch Case Action Subsystem5/1(In1)
  In6/1 -> Switch Case Action Subsystem4/1(In1)
  In5/1 -> Switch Case Action Subsystem3/1(In1)
  In4/1 -> Switch Case Action Subsystem2/1(In1)
  In3/1 -> Switch Case Action Subsystem1/1(In1)
  In2/1 -> Switch Case Action Subsystem/1(In1)
  Switch Case/10 -> Switch Case Action Subsystem9/Action
  Switch Case/9 -> Switch Case Action Subsystem8/Action
  Switch Case/8 -> Switch Case Action Subsystem6/Action
  Switch Case Action Subsystem9/1(Out1) -> Merge/10
  Switch Case Action Subsystem8/1(Out1) -> Merge/9
  Switch Case Action Subsystem6/1(Out1) -> Merge/8
  Switch Case/7 -> Switch Case Action Subsystem7/Action
  Switch Case/1 -> Switch Case Action Subsystem/Action
  Switch Case/2 -> Switch Case Action Subsystem1/Action
  Switch Case/3 -> Switch Case Action Subsystem2/Action
  Switch Case/4 -> Switch Case Action Subsystem3/Action
  Switch Case/5 -> Switch Case Action Subsystem4/Action
  Switch Case Action Subsystem/1(Out1) -> Merge/1
  Switch Case Action Subsystem1/1(Out1) -> Merge/2
  Switch Case Action Subsystem2/1(Out1) -> Merge/3
  Switch Case Action Subsystem3/1(Out1) -> Merge/4
  Switch Case Action Subsystem4/1(Out1) -> Merge/5
  Merge/1 -> data/1
  case/1 -> Switch Case/1
  Switch Case Action Subsystem7/1(Out1) -> Merge/7
  Switch Case Action Subsystem5/1(Out1) -> Merge/6
  Switch Case/6 -> Switch Case Action Subsystem5/Action

== system uwb_hw_cosim_kintex/Subsystem2/Creat n_re/delay transmition/Truyen Tre don vi ==
  case : Inport
  In2 : Inport  Port=2
  In3 : Inport  Port=3
  In4 : Inport  Port=4
  In5 : Inport  Port=5
  In6 : Inport  Port=6
  In7 : Inport  Port=7
  In8 : Inport  Port=8
  In9 : Inport  Port=9
  In10 : Inport  Port=10
  In11 : Inport  Port=11
  Merge : Merge  Inputs=10
  Switch Case : SwitchCase  CaseConditions={1,2,3,4,5,6,7,8,9}
  Switch Case Action Subsystem : Subsystem  TreatAsAtomicUnit=on
      mask Display: disp('case 1')
  Switch Case Action Subsystem1 : Subsystem  TreatAsAtomicUnit=on
      mask Display: disp('case 2')
  Switch Case Action Subsystem2 : Subsystem  TreatAsAtomicUnit=on
      mask Display: disp('case 3')
  Switch Case Action Subsystem3 : Subsystem  TreatAsAtomicUnit=on
      mask Display: disp('case 4')
  Switch Case Action Subsystem4 : Subsystem  TreatAsAtomicUnit=on
      mask Display: disp('case 5')
  Switch Case Action Subsystem5 : Subsystem  TreatAsAtomicUnit=on
      mask Display: disp('case 6')
  Switch Case Action Subsystem6 : Subsystem  TreatAsAtomicUnit=on
      mask Display: disp('case 8')
  Switch Case Action Subsystem7 : Subsystem  TreatAsAtomicUnit=on
      mask Display: disp('case 7')
  Switch Case Action Subsystem8 : Subsystem  TreatAsAtomicUnit=on
      mask Display: disp('case 9')
  Switch Case Action Subsystem9 : Subsystem  TreatAsAtomicUnit=on
      mask Display: disp('case 10')
  data : Outport
  wires:
  Switch Case/6 -> Switch Case Action Subsystem5/Action
  Switch Case Action Subsystem5/1(Out1) -> Merge/6
  Switch Case Action Subsystem7/1(Out1) -> Merge/7
  case/1 -> Switch Case/1
  Merge/1 -> data/1
  Switch Case Action Subsystem4/1(Out1) -> Merge/5
  Switch Case Action Subsystem3/1(Out1) -> Merge/4
  Switch Case Action Subsystem2/1(Out1) -> Merge/3
  Switch Case Action Subsystem1/1(Out1) -> Merge/2
  Switch Case Action Subsystem/1(Out1) -> Merge/1
  Switch Case/5 -> Switch Case Action Subsystem4/Action
  Switch Case/4 -> Switch Case Action Subsystem3/Action
  Switch Case/3 -> Switch Case Action Subsystem2/Action
  Switch Case/2 -> Switch Case Action Subsystem1/Action
  Switch Case/1 -> Switch Case Action Subsystem/Action
  Switch Case/7 -> Switch Case Action Subsystem7/Action
  Switch Case Action Subsystem6/1(Out1) -> Merge/8
  Switch Case Action Subsystem8/1(Out1) -> Merge/9
  Switch Case Action Subsystem9/1(Out1) -> Merge/10
  Switch Case/8 -> Switch Case Action Subsystem6/Action
  Switch Case/9 -> Switch Case Action Subsystem8/Action
  Switch Case/10 -> Switch Case Action Subsystem9/Action
  In2/1 -> Switch Case Action Subsystem/1(In1)
  In3/1 -> Switch Case Action Subsystem1/1(In1)
  In4/1 -> Switch Case Action Subsystem2/1(In1)
  In5/1 -> Switch Case Action Subsystem3/1(In1)
  In6/1 -> Switch Case Action Subsystem4/1(In1)
  In7/1 -> Switch Case Action Subsystem5/1(In1)
  In8/1 -> Switch Case Action Subsystem7/1(In1)
  In9/1 -> Switch Case Action Subsystem6/1(In1)
  In10/1 -> Switch Case Action Subsystem8/1(In1)
  In11/1 -> Switch Case Action Subsystem9/1(In1)

== system uwb_hw_cosim_kintex/Subsystem2/Creat n_re/delay transmition/Truyen Tre tram ==
  case : Inport
  In2 : Inport  Port=2
  In3 : Inport  Port=3
  In4 : Inport  Port=4
  In5 : Inport  Port=5
  In6 : Inport  Port=6
  In7 : Inport  Port=7
  In8 : Inport  Port=8
  In9 : Inport  Port=9
  In10 : Inport  Port=10
  In11 : Inport  Port=11
  Merge : Merge  Inputs=10
  Switch Case : SwitchCase  CaseConditions={1,2,3,4,5,6,7,8,9}
  Switch Case Action Subsystem : Subsystem  TreatAsAtomicUnit=on
      mask Display: disp('case 1')
  Switch Case Action Subsystem1 : Subsystem  TreatAsAtomicUnit=on
      mask Display: disp('case 2')
  Switch Case Action Subsystem2 : Subsystem  TreatAsAtomicUnit=on
      mask Display: disp('case 3')
  Switch Case Action Subsystem3 : Subsystem  TreatAsAtomicUnit=on
      mask Display: disp('case 4')
  Switch Case Action Subsystem4 : Subsystem  TreatAsAtomicUnit=on
      mask Display: disp('case 5')
  Switch Case Action Subsystem5 : Subsystem  TreatAsAtomicUnit=on
      mask Display: disp('case 6')
  Switch Case Action Subsystem6 : Subsystem  TreatAsAtomicUnit=on
      mask Display: disp('case 8')
  Switch Case Action Subsystem7 : Subsystem  TreatAsAtomicUnit=on
      mask Display: disp('case 7')
  Switch Case Action Subsystem8 : Subsystem  TreatAsAtomicUnit=on
      mask Display: disp('case 9')
  Switch Case Action Subsystem9 : Subsystem  TreatAsAtomicUnit=on
      mask Display: disp('case 10')
  data : Outport
  wires:
  Switch Case/6 -> Switch Case Action Subsystem5/Action
  Switch Case Action Subsystem5/1(Out1) -> Merge/6
  Switch Case Action Subsystem7/1(Out1) -> Merge/7
  case/1 -> Switch Case/1
  Merge/1 -> data/1
  Switch Case Action Subsystem4/1(Out1) -> Merge/5
  Switch Case Action Subsystem3/1(Out1) -> Merge/4
  Switch Case Action Subsystem2/1(Out1) -> Merge/3
  Switch Case Action Subsystem1/1(Out1) -> Merge/2
  Switch Case Action Subsystem/1(Out1) -> Merge/1
  Switch Case/5 -> Switch Case Action Subsystem4/Action
  Switch Case/4 -> Switch Case Action Subsystem3/Action
  Switch Case/3 -> Switch Case Action Subsystem2/Action
  Switch Case/2 -> Switch Case Action Subsystem1/Action
  Switch Case/1 -> Switch Case Action Subsystem/Action
  Switch Case/7 -> Switch Case Action Subsystem7/Action
  Switch Case Action Subsystem6/1(Out1) -> Merge/8
  Switch Case Action Subsystem8/1(Out1) -> Merge/9
  Switch Case Action Subsystem9/1(Out1) -> Merge/10
  Switch Case/8 -> Switch Case Action Subsystem6/Action
  Switch Case/9 -> Switch Case Action Subsystem8/Action
  Switch Case/10 -> Switch Case Action Subsystem9/Action
  In2/1 -> Switch Case Action Subsystem/1(In1)
  In3/1 -> Switch Case Action Subsystem1/1(In1)
  In4/1 -> Switch Case Action Subsystem2/1(In1)
  In5/1 -> Switch Case Action Subsystem3/1(In1)
  In6/1 -> Switch Case Action Subsystem4/1(In1)
  In7/1 -> Switch Case Action Subsystem5/1(In1)
  In8/1 -> Switch Case Action Subsystem7/1(In1)
  In9/1 -> Switch Case Action Subsystem6/1(In1)
  In10/1 -> Switch Case Action Subsystem8/1(In1)
  In11/1 -> Switch Case Action Subsystem9/1(In1)

== system uwb_hw_cosim_kintex/Subsystem2/Creat n_re/delay transmition/hang chuc ==
  In1 : Inport
  Integer Delay : Delay  DelayLength=10
  Integer Delay1 : Delay  DelayLength=20
  Integer Delay2 : Delay  DelayLength=30
  Integer Delay3 : Delay  DelayLength=40
  Integer Delay4 : Delay  DelayLength=50
  Integer Delay5 : Delay  DelayLength=60
  Integer Delay6 : Delay  DelayLength=70
  Integer Delay7 : Delay  DelayLength=80
  Integer Delay8 : Delay  DelayLength=90
  Out1 : Outport
  Out2 : Outport  Port=2
  Out3 : Outport  Port=3
  Out4 : Outport  Port=4
  Out5 : Outport  Port=5
  Out6 : Outport  Port=6
  Out7 : Outport  Port=7
  Out8 : Outport  Port=8
  Out9 : Outport  Port=9
  Out10 : Outport  Port=10
  wires:
  In1/1 -> Integer Delay7/1, Integer Delay8/1, Integer Delay6/1, Integer Delay5/1, Integer Delay4/1, Integer Delay3/1, Integer Delay2/1, Integer Delay1/1, Out1/1, Integer Delay/1
  Integer Delay/1 -> Out2/1
  Integer Delay1/1 -> Out3/1
  Integer Delay2/1 -> Out4/1
  Integer Delay3/1 -> Out5/1
  Integer Delay4/1 -> Out6/1
  Integer Delay5/1 -> Out7/1
  Integer Delay6/1 -> Out8/1
  Integer Delay7/1 -> Out9/1
  Integer Delay8/1 -> Out10/1

== system uwb_hw_cosim_kintex/Subsystem2/Creat n_re/delay transmition/hang don vi ==
  In1 : Inport
  Integer Delay : Delay  DelayLength=1
  Integer Delay1 : Delay
  Integer Delay2 : Delay  DelayLength=3
  Integer Delay3 : Delay  DelayLength=4
  Integer Delay4 : Delay  DelayLength=5
  Integer Delay5 : Delay  DelayLength=6
  Integer Delay6 : Delay  DelayLength=7
  Integer Delay7 : Delay  DelayLength=8
  Integer Delay8 : Delay  DelayLength=9
  Out1 : Outport
  Out2 : Outport  Port=2
  Out3 : Outport  Port=3
  Out4 : Outport  Port=4
  Out5 : Outport  Port=5
  Out6 : Outport  Port=6
  Out7 : Outport  Port=7
  Out8 : Outport  Port=8
  Out9 : Outport  Port=9
  Out10 : Outport  Port=10
  wires:
  In1/1 -> Integer Delay7/1, Integer Delay8/1, Integer Delay6/1, Integer Delay5/1, Integer Delay4/1, Integer Delay3/1, Integer Delay2/1, Integer Delay1/1, Out1/1, Integer Delay/1
  Integer Delay/1 -> Out2/1
  Integer Delay1/1 -> Out3/1
  Integer Delay2/1 -> Out4/1
  Integer Delay3/1 -> Out5/1
  Integer Delay4/1 -> Out6/1
  Integer Delay5/1 -> Out7/1
  Integer Delay6/1 -> Out8/1
  Integer Delay7/1 -> Out9/1
  Integer Delay8/1 -> Out10/1

== system uwb_hw_cosim_kintex/Subsystem2/Creat n_re/delay transmition/hang nghin ==
  In1 : Inport
  Out1 : Outport
  Out2 : Outport  Port=2
  wires:
  In1/1 -> Out1/1, Out2/1
